simulink subsystem "Copy_of_Guide_Flight_Path_Energy"  (R2025b)
settings: Solver=VariableStepAuto  StartTime=0.0  StopTime=10.0  RelTol=1e-3
undefined symbols (not defined in the file): alpha, EngineThrustCMD, Kd_alt, Ki_alt, Kp_alt, PitchIntegLim, U1
libraries: simulink_extras x5
settings Model: Creator=invrt  LastModifiedBy=angelespinoza

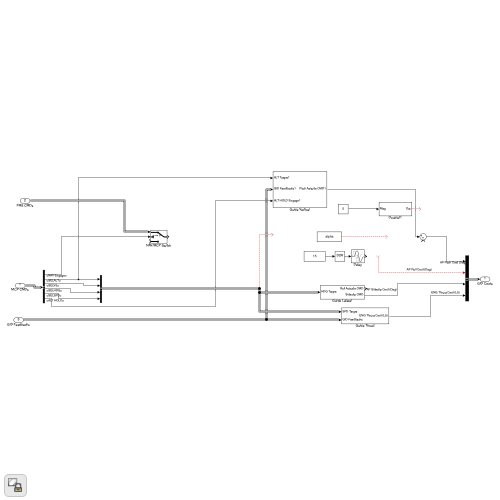
[thumbnail: Simulink's stored preview of the top-level diagram]
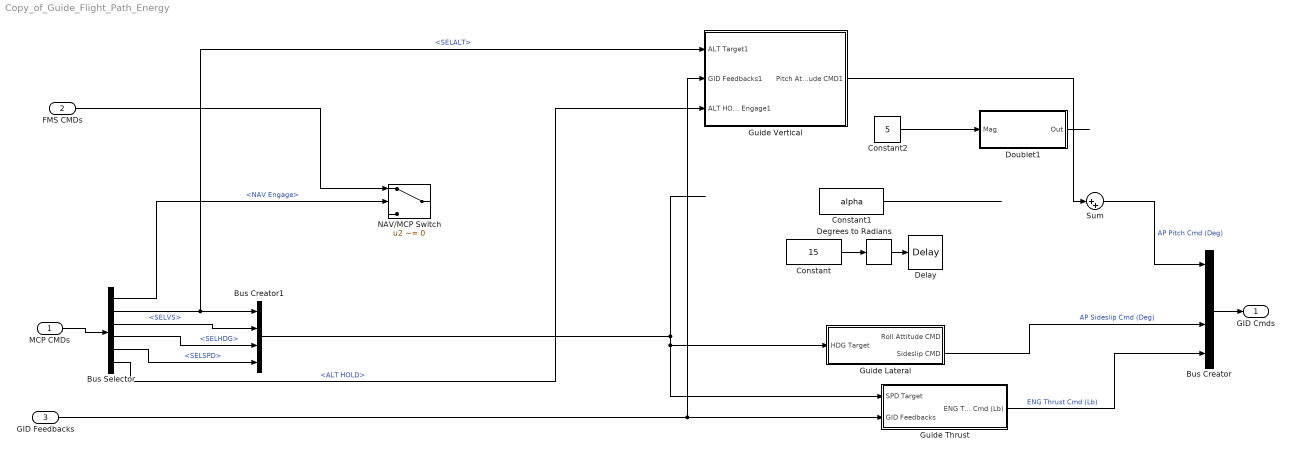
== system Copy_of_Guide_Flight_Path_Energy ==
  MCP CMDs : Inport
  FMS CMDs : Inport  Port=2
  GID Feedbacks : Inport  Port=3
  Bus Creator : BusCreator  Inputs=4
  Bus Creator1 : BusCreator  Inputs=4
  Bus Selector : BusSelector  OutputSignals=NAV Engage,Vert GID Bus.SELALT,Vert GID Bus.SELVS,Lat GID Bus.SELHDG,Spd/Mach GID Bus.SELSPD,Vert GID Bus.ALT HOLD
  Constant : Constant  Value=15
  Constant1 : Constant  Value=alpha
  Constant2 : Constant  Value=5
  Degrees to Radians : simulink_extras/Transformations/Degrees to Radians
  Delay : TransportDelay  DelayTime=5
  Doublet1 : Subsystem
  Guide Lateral : Subsystem
  Guide Thrust : Subsystem
  Guide Vertical : Subsystem
  NAV/MCP Switch : Switch  Criteria=u2 ~= 0  OutDataTypeStr=Inherit: Inherit via back propagation  SaturateOnIntegerOverflow=off
  Sum : Sum  Inputs=|++
  GID Cmds : Outport
  wires:
  Guide Lateral/2(Sideslip CMD) -> Bus Creator/3  "AP Sideslip Cmd (Deg)"
  Bus Creator/1 -> GID Cmds/1
  MCP CMDs/1 -> Bus Selector/1
  Bus Selector/1 -> NAV/MCP Switch/2  "<NAV Engage>"
  Bus Selector/2 -> Bus Creator1/1, Guide Vertical/1(ALT Target1)  "<SELALT>"
  Bus Selector/3 -> Bus Creator1/2  "<SELVS>"
  Bus Selector/4 -> Bus Creator1/3  "<SELHDG>"
  FMS CMDs/1 -> NAV/MCP Switch/1
  Bus Creator1/1 -> Guide Thrust/1(SPD Target), Guide Lateral/1(HDG Target)
  GID Feedbacks/1 -> Guide Thrust/2(GID Feedbacks), Guide Vertical/2(GID Feedbacks1)
  Guide Thrust/1(ENG Thrust Cmd (Lb)) -> Bus Creator/4  "ENG Thrust Cmd (Lb)"
  Bus Selector/5 -> Bus Creator1/4  "<SELSPD>"
  Degrees to Radians/1 -> Delay/1
  Constant/1 -> Degrees to Radians/1
  Constant2/1 -> Doublet1/1(Mag)
  Doublet1/1(Out) -> ?
  Sum/1 -> Bus Creator/1  "AP Pitch Cmd (Deg)"
  Constant1/1 -> ?
  ? -> Bus Creator/2  "AP Roll Cmd (Deg)"
  Guide Vertical/1(Pitch Attitude CMD1) -> Sum/1
  Bus Selector/6 -> Guide Vertical/3(ALT HOLD Engage1)  "<ALT HOLD>"

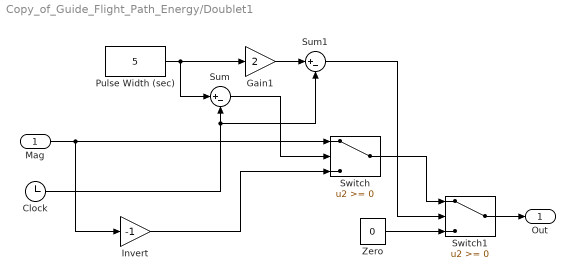
== system Copy_of_Guide_Flight_Path_Energy/Doublet1 ==
  Mag : Inport
  Clock : Clock
  Gain1 : Gain  Gain=2
  Invert : Gain  Gain=-1
  Pulse Width (sec) : Constant  Value=5
  Sum : Sum  Inputs=|+-
  Sum1 : Sum  Inputs=|+-
  Switch : Switch  SaturateOnIntegerOverflow=off  InputSameDT=off
  Switch1 : Switch  SaturateOnIntegerOverflow=off  InputSameDT=off
  Zero : Constant  Value=0
  Out : Outport
  wires:
  Sum1/1 -> Switch1/2
  Gain1/1 -> Sum1/1
  Switch1/1 -> Out/1
  Sum/1 -> Switch/2
  Clock/1 -> Sum/2, Sum1/2
  Zero/1 -> Switch1/3
  Switch/1 -> Switch1/1
  Invert/1 -> Switch/3
  Pulse Width (sec)/1 -> Gain1/1, Sum/1
  Mag/1 -> Invert/1, Switch/1

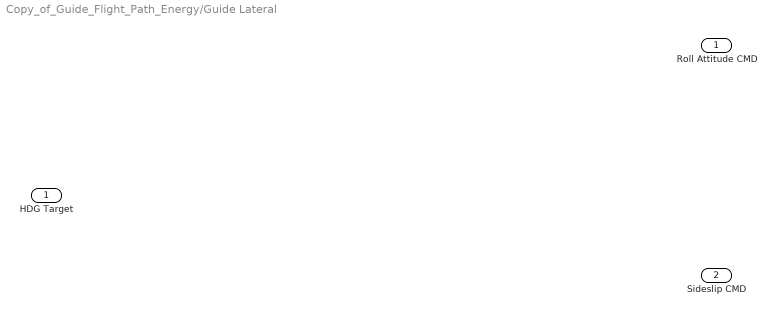
== system Copy_of_Guide_Flight_Path_Energy/Guide Lateral ==
  HDG Target : Inport
  Roll Attitude CMD : Outport
  Sideslip CMD : Outport  Port=2

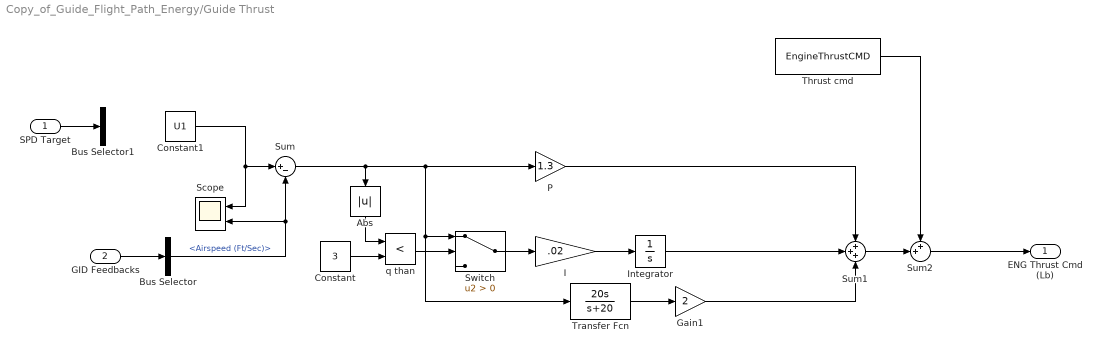
== system Copy_of_Guide_Flight_Path_Energy/Guide Thrust ==
  SPD Target : Inport
  GID Feedbacks : Inport  Port=2
  Abs : Abs  SaturateOnIntegerOverflow=off
  Bus Selector : BusSelector  OutputSignals=Airspeed (Ft/Sec)
  Bus Selector1 : BusSelector  OutputSignals=SELSPD
  Constant : Constant  Value=3
  Constant1 : Constant  Value=U1
  Gain1 : Gain  Gain=2
  I : Gain  Gain=.02
  Integrator : Integrator  LimitOutput=on  UpperSaturationLimit=1  LowerSaturationLimit=-1
  P : Gain  Gain=1.3
  Scope : Scope  NumInputPorts=2
      settings: ActiveDisplayYMinimum=868.72685468796908  ActiveDisplayYMaximum=899.17143805629928  DataLoggingVariableName=ScopeData26
  Sum : Sum  Inputs=|+-
  Sum1 : Sum  Inputs=+++
  Sum2 : Sum  Inputs=++|
  Switch : Switch  Criteria=u2 > Threshold  SaturateOnIntegerOverflow=off  InputSameDT=off
  Thrust cmd : Constant  Value=EngineThrustCMD
  Transfer Fcn : TransferFcn  Numerator=[20 0]  Denominator=[1 20]
  q than : RelationalOperator  Operator=<  OutDataTypeStr=boolean  RndMeth=Simplest  InputSameDT=off
  ENG Thrust Cmd (Lb) : Outport
  wires:
  Integrator/1 -> Sum1/2
  Gain1/1 -> Sum1/3
  Transfer Fcn/1 -> Gain1/1
  I/1 -> Integrator/1
  Abs/1 -> q than/1
  Switch/1 -> I/1
  Constant/1 -> q than/2
  q than/1 -> Switch/2
  Sum/1 -> Abs/1, P/1, Switch/1, Transfer Fcn/1
  Sum2/1 -> ENG Thrust Cmd (Lb)/1
  Thrust cmd/1 -> Sum2/1
  P/1 -> Sum1/1
  Bus Selector/1 -> Scope/2, Sum/2  "<Airspeed (Ft/Sec)>"
  GID Feedbacks/1 -> Bus Selector/1
  SPD Target/1 -> Bus Selector1/1
  Sum1/1 -> Sum2/2
  Constant1/1 -> Scope/1, Sum/1

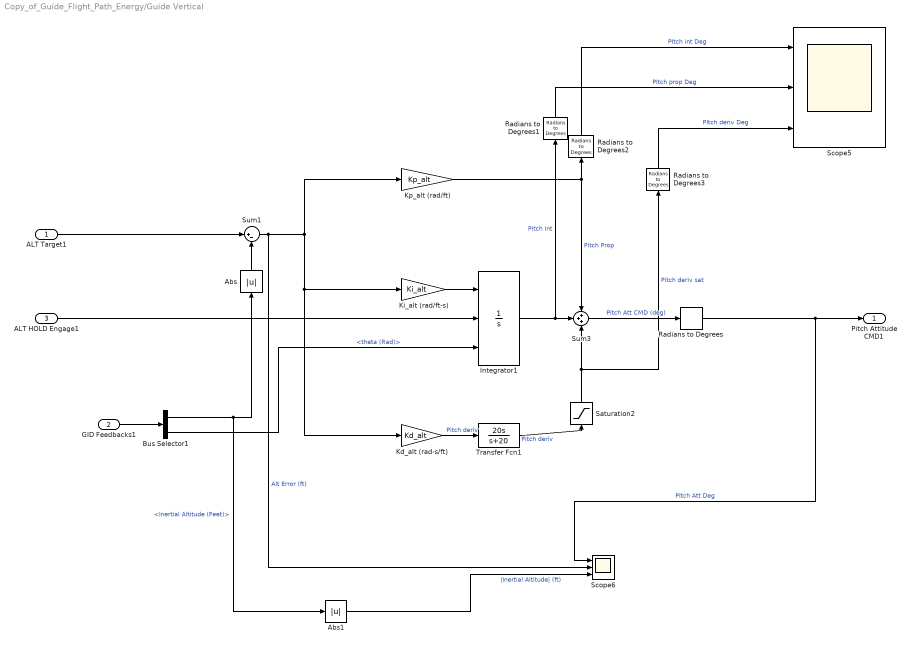
== system Copy_of_Guide_Flight_Path_Energy/Guide Vertical ==
  ALT Target1 : Inport
  GID Feedbacks1 : Inport  Port=2
  ALT HOLD Engage1 : Inport  Port=3
  " Ki_alt (rad/ft-s)" : Gain  Gain=Ki_alt
  Abs : Abs  SaturateOnIntegerOverflow=off
  Abs1 : Abs  SaturateOnIntegerOverflow=off
  Bus Selector1 : BusSelector  OutputSignals=Trans.Inertial Pos.Inertial Altitude (Feet),Rotat.Attitude.theta (Rad)
  Integrator1 : Integrator  ExternalReset=rising  InitialConditionSource=external  LimitOutput=on  UpperSaturationLimit=PitchIntegLim  LowerSaturationLimit=-PitchIntegLim
  Kd_alt (rad-s/ft) : Gain  Gain=Kd_alt
  Kp_alt (rad/ft) : Gain  Gain=Kp_alt
  Radians to Degrees{,1..3} (4 alike) : simulink_extras/Transformations/Radians to Degrees
  Saturation2 : Saturate  UpperLimit=0.2  LowerLimit=-0.2
  Scope5 : Scope  NumInputPorts=3
      settings: ActiveDisplayYMinimum=-0.26617575704278174  ActiveDisplayYMaximum=0.91199146982936086  DataLoggingVariableName=ScopeData4
  Scope6 : Scope  NumInputPorts=3
      settings: ActiveDisplayYMinimum=1.3555847553849334  ActiveDisplayYMaximum=16.242995456202713  DataLoggingVariableName=ScopeData5
  Sum1 : Sum  Inputs=|+-
  Sum3 : Sum  Inputs=+++
  Transfer Fcn1 : TransferFcn  Numerator=[20 0]  Denominator=[1 20]
  Pitch Attitude CMD1 : Outport
  wires:
  Radians to Degrees3/1 -> Scope5/3  "PItch deriv Deg"
  Radians to Degrees2/1 -> Scope5/1  "PItch int Deg"
  Radians to Degrees1/1 -> Scope5/2  "PItch prop Deg"
  Saturation2/1 -> Sum3/3, Radians to Degrees3/1  "Pitch deriv sat"
  Radians to Degrees/1 -> Pitch Attitude CMD1/1, Scope6/1  "PItch Att Deg"
  Sum3/1 -> Radians to Degrees/1  "Pitch Att CMD (deg)"
  Bus Selector1/2 -> Integrator1/3  "<theta (Rad)>"
  Abs1/1 -> Scope6/3  "|Inertial Altitude| (ft)"
  " Ki_alt (rad/ft-s)"/1 -> Integrator1/1
  Transfer Fcn1/1 -> Saturation2/1  "Pitch deriv"
  Bus Selector1/1 -> Abs/1, Abs1/1  "<Inertial Altitude (Feet)>"
  GID Feedbacks1/1 -> Bus Selector1/1
  Integrator1/1 -> Sum3/2, Radians to Degrees1/1  "Pitch Int"
  Sum1/1 -> Kp_alt (rad/ft)/1, " Ki_alt (rad/ft-s)"/1, Kd_alt (rad-s/ft)/1, Scope6/2  "Alt Error (ft)"
  Abs/1 -> Sum1/2
  Kd_alt (rad-s/ft)/1 -> Transfer Fcn1/1  "Pitch deriv"
  ALT HOLD Engage1/1 -> Integrator1/2
  Kp_alt (rad/ft)/1 -> Sum3/1, Radians to Degrees2/1  "Pitch Prop"
  ALT Target1/1 -> Sum1/1
